simulink library "CRYP_TM_MASTER"  (Simulink 8.6)
settings: Solver=ode45  StartTime=0.0  StopTime=10.0  RelTol=1e-3
libraries: cdsEpicsOut x44, cdsTP x11, cdsFilt x5, cdsFiltCtrl x4, cdsFunctionCall x4, CRYP_TM_MASTER x3, QPD x2, VIS_LIB x1, cdsMuxMatrix x1
(part 1 of 2)
settings Model: Creator=controls  LastModifiedBy=controls

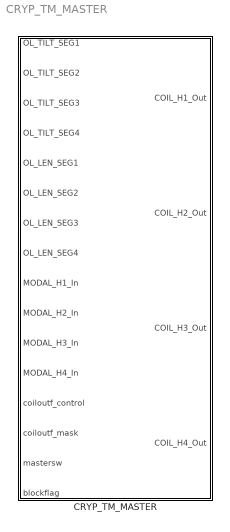
== system CRYP_TM_MASTER ==
  CRYP_TM_MASTER : Subsystem

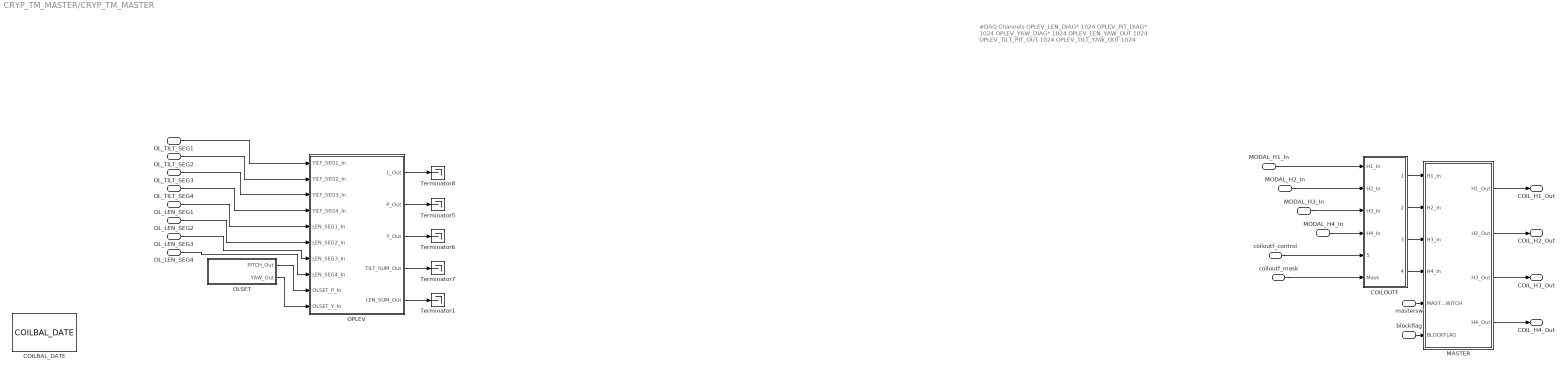
== system CRYP_TM_MASTER/CRYP_TM_MASTER ==
  note: #DAQ Channels
      | OPLEV_LEN_DIAG* 1024
      | OPLEV_PIT_DIAG* 1024
      | OPLEV_YAW_DIAG* 1024
      | OPLEV_LEN_YAW_OUT 1024
      | OPLEV_TILT_PIT_OUT 1024
      | OPLEV_TILT_YAW_OUT 1024
  OL_TILT_SEG1 : Inport
  OL_TILT_SEG2 : Inport  Port=2
  OL_TILT_SEG3 : Inport  Port=3
  OL_TILT_SEG4 : Inport  Port=4
  OL_LEN_SEG1 : Inport  Port=5
  OL_LEN_SEG2 : Inport  Port=6
  OL_LEN_SEG3 : Inport  Port=7
  OL_LEN_SEG4 : Inport  Port=8
  MODAL_H1_In : Inport  Port=9
  MODAL_H2_In : Inport  Port=10
  MODAL_H3_In : Inport  Port=11
  MODAL_H4_In : Inport  Port=12
  coiloutf_control : Inport  Port=13
  coiloutf_mask : Inport  Port=14
  mastersw : Inport  Port=15
  blockflag : Inport  Port=16
  COILBAL_DATE : VIS_LIB/COILBAL_DATE
  COILOUTF : Subsystem
  MASTER : Subsystem
  OLSET : Subsystem
  OPLEV : Subsystem
  Terminator{1,5..8} (5 alike) : Terminator
  COIL_H1_Out : Outport
  COIL_H2_Out : Outport  Port=2
  COIL_H3_Out : Outport  Port=3
  COIL_H4_Out : Outport  Port=4
  wires:
  MODAL_H4_In/1 -> COILOUTF/4(H4_In)
  MODAL_H3_In/1 -> COILOUTF/3(H3_In)
  MODAL_H2_In/1 -> COILOUTF/2(H2_In)
  MODAL_H1_In/1 -> COILOUTF/1(H1_In)
  OL_TILT_SEG3/1 -> OPLEV/3(TILT_SEG3_In)
  OL_LEN_SEG4/1 -> OPLEV/8(LEN_SEG4_In)
  OL_LEN_SEG3/1 -> OPLEV/7(LEN_SEG3_In)
  OL_LEN_SEG2/1 -> OPLEV/6(LEN_SEG2_In)
  OL_LEN_SEG1/1 -> OPLEV/5(LEN_SEG1_In)
  OL_TILT_SEG4/1 -> OPLEV/4(TILT_SEG4_In)
  OL_TILT_SEG2/1 -> OPLEV/2(TILT_SEG2_In)
  OL_TILT_SEG1/1 -> OPLEV/1(TILT_SEG1_In)
  COILOUTF/4(H4_Out) -> MASTER/4(H4_In)
  COILOUTF/3(H3_Out) -> MASTER/3(H3_In)
  COILOUTF/2(H2_Out) -> MASTER/2(H2_In)
  COILOUTF/1(H1_Out) -> MASTER/1(H1_In)
  MASTER/1(H1_Out) -> COIL_H1_Out/1
  MASTER/2(H2_Out) -> COIL_H2_Out/1
  MASTER/3(H3_Out) -> COIL_H3_Out/1
  MASTER/4(H4_Out) -> COIL_H4_Out/1
  OLSET/1(PITCH_Out) -> OPLEV/9(OLSET_P_In)
  OLSET/2(YAW_Out) -> OPLEV/10(OLSET_Y_In)
  coiloutf_control/1 -> COILOUTF/5(Control)
  coiloutf_mask/1 -> COILOUTF/6(Mask)
  mastersw/1 -> MASTER/5(MASTERSWITCH)
  blockflag/1 -> MASTER/6(BLOCKFLAG)
  OPLEV/1(L_Out) -> Terminator8/1
  OPLEV/2(P_Out) -> Terminator5/1
  OPLEV/3(Y_Out) -> Terminator6/1
  OPLEV/4(TILT_SUM_Out) -> Terminator7/1
  OPLEV/5(LEN_SUM_Out) -> Terminator1/1

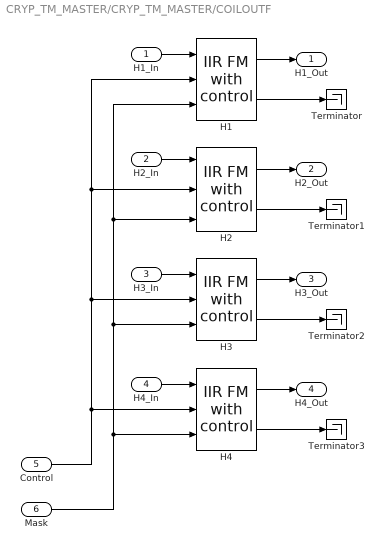
== system CRYP_TM_MASTER/CRYP_TM_MASTER/COILOUTF ==
  H1_In : Inport
  H2_In : Inport  Port=2
  H3_In : Inport  Port=3
  H4_In : Inport  Port=4
  Control : Inport  Port=5
  Mask : Inport  Port=6
  H1 : cdsFiltCtrl/IIR FM with control  Tag=cdsFiltCtrl  Description=|
      | cdsFiltCntrl is the standard IIR filter module (exactly the same as cdsFilt) but with added control data output 'Ctrl'. Filter module digital signal output appears on the first output, which is called 'Val'. 'Ctrl' output has a bit pattern encoding the state of filter's on/off switches (FM1 through FM10). The bit values are:
      |                                                                                                                                                                                                                                                                                                                                       
      | module 	hex	dec                                                                                                                                                                                                                                                                                                                       
      | -----------------------                                                                                                                                                                                                                                                                                                               
      | FM1	0x20                    32                                                                                                                                                                                                                                                                                                        
      | FM2	0x80                     128                                                                                                                                                                                                                                                                                                      
      | FM3	0x200                   512                                                                                                                                                                                                                                                                                                       
      | FM4	0x800                   2048                                                                                                                                                                                                                                                                                                      
      | FM5	0x2000                 8192                                                                                                                                                                                                                                                                                                       
      | FM6	0x8000                 32768                                                                                                                                                                                                                                                                                                      
      | FM7	0x20000                131072                                                                                                                                                                                                                                                                                                     
      | FM8	0x80000                 524288                                                                                                                                                                                                                                                                                                    
      | FM9	0x200000               2097152                                                                                                                                                                                                                                                                                                    
      | FM10	0x800000               8388608                                                                                                                                                                                                                                                                                                   
      |                                                                                                                                                                                                                                                                                                                                       
      | This bit data can be used to drive some other switches or it can be output using a binary I/O module.
      settings: AttributesFormatString=%<Tag>
  H2 : cdsFiltCtrl/IIR FM with control  Tag=cdsFiltCtrl  Description=|
      | cdsFiltCntrl is the standard IIR filter module (exactly the same as cdsFilt) but with added control data output 'Ctrl'. Filter module digital signal output appears on the first output, which is called 'Val'. 'Ctrl' output has a bit pattern encoding the state of filter's on/off switches (FM1 through FM10). The bit values are:
      |                                                                                                                                                                                                                                                                                                                                       
      | module 	hex	dec                                                                                                                                                                                                                                                                                                                       
      | -----------------------                                                                                                                                                                                                                                                                                                               
      | FM1	0x20                    32                                                                                                                                                                                                                                                                                                        
      | FM2	0x80                     128                                                                                                                                                                                                                                                                                                      
      | FM3	0x200                   512                                                                                                                                                                                                                                                                                                       
      | FM4	0x800                   2048                                                                                                                                                                                                                                                                                                      
      | FM5	0x2000                 8192                                                                                                                                                                                                                                                                                                       
      | FM6	0x8000                 32768                                                                                                                                                                                                                                                                                                      
      | FM7	0x20000                131072                                                                                                                                                                                                                                                                                                     
      | FM8	0x80000                 524288                                                                                                                                                                                                                                                                                                    
      | FM9	0x200000               2097152                                                                                                                                                                                                                                                                                                    
      | FM10	0x800000               8388608                                                                                                                                                                                                                                                                                                   
      |                                                                                                                                                                                                                                                                                                                                       
      | This bit data can be used to drive some other switches or it can be output using a binary I/O module.
      settings: AttributesFormatString=%<Tag>
  H3 : cdsFiltCtrl/IIR FM with control  Tag=cdsFiltCtrl  Description=|
      | cdsFiltCntrl is the standard IIR filter module (exactly the same as cdsFilt) but with added control data output 'Ctrl'. Filter module digital signal output appears on the first output, which is called 'Val'. 'Ctrl' output has a bit pattern encoding the state of filter's on/off switches (FM1 through FM10). The bit values are:
      |                                                                                                                                                                                                                                                                                                                                       
      | module 	hex	dec                                                                                                                                                                                                                                                                                                                       
      | -----------------------                                                                                                                                                                                                                                                                                                               
      | FM1	0x20                    32                                                                                                                                                                                                                                                                                                        
      | FM2	0x80                     128                                                                                                                                                                                                                                                                                                      
      | FM3	0x200                   512                                                                                                                                                                                                                                                                                                       
      | FM4	0x800                   2048                                                                                                                                                                                                                                                                                                      
      | FM5	0x2000                 8192                                                                                                                                                                                                                                                                                                       
      | FM6	0x8000                 32768                                                                                                                                                                                                                                                                                                      
      | FM7	0x20000                131072                                                                                                                                                                                                                                                                                                     
      | FM8	0x80000                 524288                                                                                                                                                                                                                                                                                                    
      | FM9	0x200000               2097152                                                                                                                                                                                                                                                                                                    
      | FM10	0x800000               8388608                                                                                                                                                                                                                                                                                                   
      |                                                                                                                                                                                                                                                                                                                                       
      | This bit data can be used to drive some other switches or it can be output using a binary I/O module.
      settings: AttributesFormatString=%<Tag>
  H4 : cdsFiltCtrl/IIR FM with control  Tag=cdsFiltCtrl  Description=|
      | cdsFiltCntrl is the standard IIR filter module (exactly the same as cdsFilt) but with added control data output 'Ctrl'. Filter module digital signal output appears on the first output, which is called 'Val'. 'Ctrl' output has a bit pattern encoding the state of filter's on/off switches (FM1 through FM10). The bit values are:
      |                                                                                                                                                                                                                                                                                                                                       
      | module 	hex	dec                                                                                                                                                                                                                                                                                                                       
      | -----------------------                                                                                                                                                                                                                                                                                                               
      | FM1	0x20                    32                                                                                                                                                                                                                                                                                                        
      | FM2	0x80                     128                                                                                                                                                                                                                                                                                                      
      | FM3	0x200                   512                                                                                                                                                                                                                                                                                                       
      | FM4	0x800                   2048                                                                                                                                                                                                                                                                                                      
      | FM5	0x2000                 8192                                                                                                                                                                                                                                                                                                       
      | FM6	0x8000                 32768                                                                                                                                                                                                                                                                                                      
      | FM7	0x20000                131072                                                                                                                                                                                                                                                                                                     
      | FM8	0x80000                 524288                                                                                                                                                                                                                                                                                                    
      | FM9	0x200000               2097152                                                                                                                                                                                                                                                                                                    
      | FM10	0x800000               8388608                                                                                                                                                                                                                                                                                                   
      |                                                                                                                                                                                                                                                                                                                                       
      | This bit data can be used to drive some other switches or it can be output using a binary I/O module.
      settings: AttributesFormatString=%<Tag>
  Terminator{,1..3} (4 alike) : Terminator
  H1_Out : Outport
  H2_Out : Outport  Port=2
  H3_Out : Outport  Port=3
  H4_Out : Outport  Port=4
  wires:
  H1/1 -> H1_Out/1
  H1_In/1 -> H1/1
  H2_In/1 -> H2/1
  H2/1 -> H2_Out/1
  H3_In/1 -> H3/1
  H3/1 -> H3_Out/1
  H4_In/1 -> H4/1
  H4/1 -> H4_Out/1
  H1/2 -> Terminator/1
  H2/2 -> Terminator1/1
  H4/2 -> Terminator3/1
  H3/2 -> Terminator2/1
  Mask/1 -> H4/3, H3/3, H2/3, H1/3
  Control/1 -> H4/2, H3/2, H2/2, H1/2

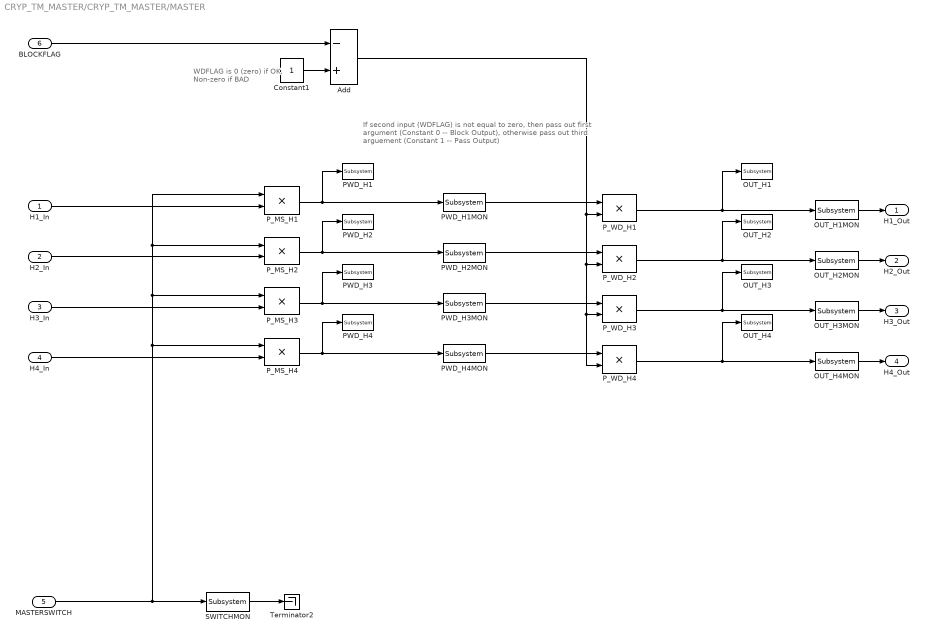
== system CRYP_TM_MASTER/CRYP_TM_MASTER/MASTER ==
  note: WDFLAG is 0 (zero) if OK,
      | Non-zero if BAD
  note: If second input (WDFLAG) is not equal to zero,
      | then pass out first argument (Constant 0 -- Block Output),
      | otherwise pass out third arguement (Constant 1 -- Pass Output)
  H1_In : Inport
  H2_In : Inport  Port=2
  H3_In : Inport  Port=3
  H4_In : Inport  Port=4
  MASTERSWITCH : Inport  Port=5
  BLOCKFLAG : Inport  Port=6
  Add : Sum  Inputs=-+
  Constant1 : Constant
  OUT_H{1..4} (4 alike) : cdsTP/Subsystem  Tag=Test Point
      settings: AttributesFormatString=%<Tag>
  OUT_H1MON : cdsEpicsOut/Subsystem  Tag=cdsEpicsOutput  Description=|
      | Purpose:                                          
      | Output a FE signal to an EPICS channel.           
      |                                                   
      | Operation:                                        
      | Takes input value and passes it to EPICS record.  
      |                                                   
      | Usage:                                            
      | Name the part with the desired EPICS rrecord name.
      settings: AttributesFormatString=%<Tag>
  OUT_H2MON : cdsEpicsOut/Subsystem  Tag=cdsEpicsOutput  Description=|
      | Purpose:                                          
      | Output a FE signal to an EPICS channel.           
      |                                                   
      | Operation:                                        
      | Takes input value and passes it to EPICS record.  
      |                                                   
      | Usage:                                            
      | Name the part with the desired EPICS rrecord name.
      settings: AttributesFormatString=%<Tag>
  OUT_H3MON : cdsEpicsOut/Subsystem  Tag=cdsEpicsOutput  Description=|
      | Purpose:                                          
      | Output a FE signal to an EPICS channel.           
      |                                                   
      | Operation:                                        
      | Takes input value and passes it to EPICS record.  
      |                                                   
      | Usage:                                            
      | Name the part with the desired EPICS rrecord name.
      settings: AttributesFormatString=%<Tag>
  OUT_H4MON : cdsEpicsOut/Subsystem  Tag=cdsEpicsOutput  Description=|
      | Purpose:                                          
      | Output a FE signal to an EPICS channel.           
      |                                                   
      | Operation:                                        
      | Takes input value and passes it to EPICS record.  
      |                                                   
      | Usage:                                            
      | Name the part with the desired EPICS rrecord name.
      settings: AttributesFormatString=%<Tag>
  PWD_H{1..4} (4 alike) : cdsTP/Subsystem  Tag=Test Point
      settings: AttributesFormatString=%<Tag>
  PWD_H1MON : cdsEpicsOut/Subsystem  Tag=cdsEpicsOutput  Description=|
      | Purpose:                                          
      | Output a FE signal to an EPICS channel.           
      |                                                   
      | Operation:                                        
      | Takes input value and passes it to EPICS record.  
      |                                                   
      | Usage:                                            
      | Name the part with the desired EPICS rrecord name.
      settings: AttributesFormatString=%<Tag>
  PWD_H2MON : cdsEpicsOut/Subsystem  Tag=cdsEpicsOutput  Description=|
      | Purpose:                                          
      | Output a FE signal to an EPICS channel.           
      |                                                   
      | Operation:                                        
      | Takes input value and passes it to EPICS record.  
      |                                                   
      | Usage:                                            
      | Name the part with the desired EPICS rrecord name.
      settings: AttributesFormatString=%<Tag>
  PWD_H3MON : cdsEpicsOut/Subsystem  Tag=cdsEpicsOutput  Description=|
      | Purpose:                                          
      | Output a FE signal to an EPICS channel.           
      |                                                   
      | Operation:                                        
      | Takes input value and passes it to EPICS record.  
      |                                                   
      | Usage:                                            
      | Name the part with the desired EPICS rrecord name.
      settings: AttributesFormatString=%<Tag>
  PWD_H4MON : cdsEpicsOut/Subsystem  Tag=cdsEpicsOutput  Description=|
      | Purpose:                                          
      | Output a FE signal to an EPICS channel.           
      |                                                   
      | Operation:                                        
      | Takes input value and passes it to EPICS record.  
      |                                                   
      | Usage:                                            
      | Name the part with the desired EPICS rrecord name.
      settings: AttributesFormatString=%<Tag>
  P_MS_H{1..4} (4 alike) : Product  RndMeth=Zero
  P_WD_H{1..4} (4 alike) : Product  RndMeth=Zero
  SWITCHMON : cdsEpicsOut/Subsystem  Tag=cdsEpicsOutput  Description=|
      | Purpose:                                          
      | Output a FE signal to an EPICS channel.           
      |                                                   
      | Operation:                                        
      | Takes input value and passes it to EPICS record.  
      |                                                   
      | Usage:                                            
      | Name the part with the desired EPICS rrecord name.
      settings: AttributesFormatString=%<Tag>
  Terminator2 : Terminator
  H1_Out : Outport
  H2_Out : Outport  Port=2
  H3_Out : Outport  Port=3
  H4_Out : Outport  Port=4
  wires:
  SWITCHMON/1 -> Terminator2/1
  BLOCKFLAG/1 -> Add/1
  Constant1/1 -> Add/2
  P_WD_H4/1 -> OUT_H4/1, OUT_H4MON/1
  P_WD_H3/1 -> OUT_H3/1, OUT_H3MON/1
  P_WD_H2/1 -> OUT_H2/1, OUT_H2MON/1
  P_WD_H1/1 -> OUT_H1/1, OUT_H1MON/1
  P_MS_H4/1 -> PWD_H4/1, PWD_H4MON/1
  P_MS_H3/1 -> PWD_H3/1, PWD_H3MON/1
  P_MS_H2/1 -> PWD_H2/1, PWD_H2MON/1
  P_MS_H1/1 -> PWD_H1/1, PWD_H1MON/1
  OUT_H4MON/1 -> H4_Out/1
  OUT_H3MON/1 -> H3_Out/1
  OUT_H1MON/1 -> H1_Out/1
  OUT_H2MON/1 -> H2_Out/1
  MASTERSWITCH/1 -> SWITCHMON/1, P_MS_H1/1, P_MS_H2/1, P_MS_H3/1, P_MS_H4/1
  H4_In/1 -> P_MS_H4/2
  H3_In/1 -> P_MS_H3/2
  H2_In/1 -> P_MS_H2/2
  H1_In/1 -> P_MS_H1/2
  PWD_H1MON/1 -> P_WD_H1/1
  PWD_H2MON/1 -> P_WD_H2/1
  PWD_H3MON/1 -> P_WD_H3/1
  PWD_H4MON/1 -> P_WD_H4/1
  Add/1 -> P_WD_H4/2, P_WD_H3/2, P_WD_H2/2, P_WD_H1/2

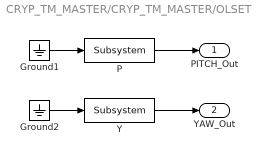
== system CRYP_TM_MASTER/CRYP_TM_MASTER/OLSET ==
  Ground1 : Ground
  Ground2 : Ground
  P : cdsFilt/Subsystem  Tag=cdsFilt  Description=|
      | Purpose:                                                                                                                                                                                                                                  
      | Standard CDS IIR filter module.                                                                                                                                                                                                           
      |                                                                                                                                                                                                                                           
      | Operation:                                                                                                                                                                                                                                
      | Consists of 10 second order section IIR filters, plus a ramped gain stage. In FE code, also provides pre-defined test points and excitation channel inputs. The filter coefficients are defined in the LIGO system using the 'foton' tool.
      |                                                                                                                                                                                                                                           
      | Usage:                                                                                                                                                                                                                                    
      | Name the part with the desired filter module name.
      settings: AttributesFormatString=%<Tag>
  Y : cdsFilt/Subsystem  Tag=cdsFilt  Description=|
      | Purpose:                                                                                                                                                                                                                                  
      | Standard CDS IIR filter module.                                                                                                                                                                                                           
      |                                                                                                                                                                                                                                           
      | Operation:                                                                                                                                                                                                                                
      | Consists of 10 second order section IIR filters, plus a ramped gain stage. In FE code, also provides pre-defined test points and excitation channel inputs. The filter coefficients are defined in the LIGO system using the 'foton' tool.
      |                                                                                                                                                                                                                                           
      | Usage:                                                                                                                                                                                                                                    
      | Name the part with the desired filter module name.
      settings: AttributesFormatString=%<Tag>
  PITCH_Out : Outport
  YAW_Out : Outport  Port=2
  wires:
  P/1 -> PITCH_Out/1
  Y/1 -> YAW_Out/1
  Ground1/1 -> P/1
  Ground2/1 -> Y/1

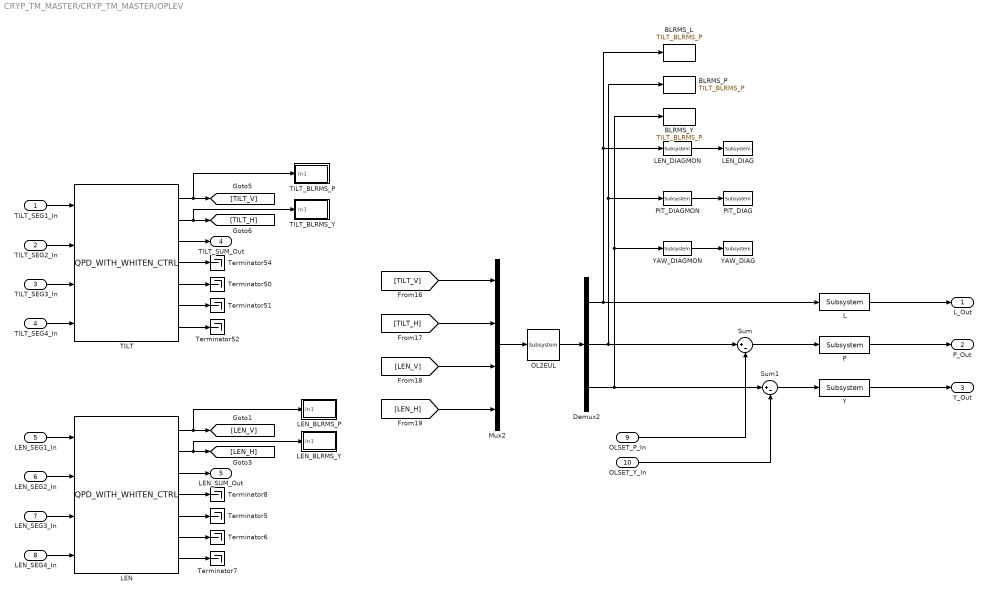
== system CRYP_TM_MASTER/CRYP_TM_MASTER/OPLEV ==
  TILT_SEG1_In : Inport
  TILT_SEG2_In : Inport  Port=2
  TILT_SEG3_In : Inport  Port=3
  TILT_SEG4_In : Inport  Port=4
  LEN_SEG1_In : Inport  Port=5
  LEN_SEG2_In : Inport  Port=6
  LEN_SEG3_In : Inport  Port=7
  LEN_SEG4_In : Inport  Port=8
  OLSET_P_In : Inport  Port=9
  OLSET_Y_In : Inport  Port=10
  BLRMS_L : CRYP_TM_MASTER/CRYP_TM_MASTER/OPLEV/TILT_BLRMS_P
  BLRMS_P : CRYP_TM_MASTER/CRYP_TM_MASTER/OPLEV/TILT_BLRMS_P
  BLRMS_Y : CRYP_TM_MASTER/CRYP_TM_MASTER/OPLEV/TILT_BLRMS_P
  Demux2 : Demux  Outputs=3
  L : cdsFilt/Subsystem  Tag=cdsFilt  Description=|
      | Purpose:                                                                                                                                                                                                                                  
      | Standard CDS IIR filter module.                                                                                                                                                                                                           
      |                                                                                                                                                                                                                                           
      | Operation:                                                                                                                                                                                                                                
      | Consists of 10 second order section IIR filters, plus a ramped gain stage. In FE code, also provides pre-defined test points and excitation channel inputs. The filter coefficients are defined in the LIGO system using the 'foton' tool.
      |                                                                                                                                                                                                                                           
      | Usage:                                                                                                                                                                                                                                    
      | Name the part with the desired filter module name.
      settings: AttributesFormatString=%<Tag>
  LEN : QPD/QPD_WITH_WHITEN_CTRL
  LEN_BLRMS_P : Subsystem
  LEN_BLRMS_Y : Subsystem
  LEN_DIAG : cdsTP/Subsystem  Tag=Test Point
      settings: AttributesFormatString=%<Tag>
  LEN_DIAGMON : cdsEpicsOut/Subsystem  Tag=cdsEpicsOutput  Description=|
      | Purpose:                                          
      | Output a FE signal to an EPICS channel.           
      |                                                   
      | Operation:                                        
      | Takes input value and passes it to EPICS record.  
      |                                                   
      | Usage:                                            
      | Name the part with the desired EPICS rrecord name.
      settings: AttributesFormatString=%<Tag>
  Mux2 : Mux
  OL2EUL : cdsMuxMatrix/Subsystem  Tag=cdsMuxMatrix  Description=Any size matrix. Inputs and outputs must be connected using Mux and Demux parts.
      settings: AttributesFormatString=%<Tag>
  P : cdsFilt/Subsystem  Tag=cdsFilt  Description=|
      | Purpose:                                                                                                                                                                                                                                  
      | Standard CDS IIR filter module.                                                                                                                                                                                                           
      |                                                                                                                                                                                                                                           
      | Operation:                                                                                                                                                                                                                                
      | Consists of 10 second order section IIR filters, plus a ramped gain stage. In FE code, also provides pre-defined test points and excitation channel inputs. The filter coefficients are defined in the LIGO system using the 'foton' tool.
      |                                                                                                                                                                                                                                           
      | Usage:                                                                                                                                                                                                                                    
      | Name the part with the desired filter module name.
      settings: AttributesFormatString=%<Tag>
  PIT_DIAG : cdsTP/Subsystem  Tag=Test Point
      settings: AttributesFormatString=%<Tag>
  PIT_DIAGMON : cdsEpicsOut/Subsystem  Tag=cdsEpicsOutput  Description=|
      | Purpose:                                          
      | Output a FE signal to an EPICS channel.           
      |                                                   
      | Operation:                                        
      | Takes input value and passes it to EPICS record.  
      |                                                   
      | Usage:                                            
      | Name the part with the desired EPICS rrecord name.
      settings: AttributesFormatString=%<Tag>
  Sum : Sum  Inputs=|+-
  Sum1 : Sum  Inputs=|+-
  TILT : QPD/QPD_WITH_WHITEN_CTRL
  TILT_BLRMS_P : Subsystem
  TILT_BLRMS_Y : Subsystem
  Terminator{5..8,50..52,54} (8 alike) : Terminator
  Y : cdsFilt/Subsystem  Tag=cdsFilt  Description=|
      | Purpose:                                                                                                                                                                                                                                  
      | Standard CDS IIR filter module.                                                                                                                                                                                                           
      |                                                                                                                                                                                                                                           
      | Operation:                                                                                                                                                                                                                                
      | Consists of 10 second order section IIR filters, plus a ramped gain stage. In FE code, also provides pre-defined test points and excitation channel inputs. The filter coefficients are defined in the LIGO system using the 'foton' tool.
      |                                                                                                                                                                                                                                           
      | Usage:                                                                                                                                                                                                                                    
      | Name the part with the desired filter module name.
      settings: AttributesFormatString=%<Tag>
  YAW_DIAG : cdsTP/Subsystem  Tag=Test Point
      settings: AttributesFormatString=%<Tag>
  YAW_DIAGMON : cdsEpicsOut/Subsystem  Tag=cdsEpicsOutput  Description=|
      | Purpose:                                          
      | Output a FE signal to an EPICS channel.           
      |                                                   
      | Operation:                                        
      | Takes input value and passes it to EPICS record.  
      |                                                   
      | Usage:                                            
      | Name the part with the desired EPICS rrecord name.
      settings: AttributesFormatString=%<Tag>
  L_Out : Outport
  P_Out : Outport  Port=2
  Y_Out : Outport  Port=3
  TILT_SUM_Out : Outport  Port=4
  LEN_SUM_Out : Outport  Port=5
  wires:
  [TILT_H] -> Mux2/2
  Demux2/3 -> Sum1/1, BLRMS_Y/1, YAW_DIAGMON/1
  LEN/4 -> Terminator8/1
  LEN/5 -> Terminator5/1
  LEN/6 -> Terminator6/1
  LEN/7 -> Terminator7/1
  [TILT_V] -> Mux2/1
  LEN_SEG4_In/1 -> LEN/4
  LEN/2 -> [LEN_H], LEN_BLRMS_Y/1(In1)
  LEN/1 -> [LEN_V], LEN_BLRMS_P/1(In1)
  LEN/3 -> LEN_SUM_Out/1
  [LEN_V] -> Mux2/3
  LEN_SEG1_In/1 -> LEN/1
  LEN_SEG2_In/1 -> LEN/2
  LEN_SEG3_In/1 -> LEN/3
  OL2EUL/1 -> Demux2/1
  TILT_SEG1_In/1 -> TILT/1
  TILT_SEG2_In/1 -> TILT/2
  TILT_SEG3_In/1 -> TILT/3
  TILT_SEG4_In/1 -> TILT/4
  TILT/2 -> TILT_BLRMS_Y/1(In1), [TILT_H]
  TILT/1 -> TILT_BLRMS_P/1(In1), [TILT_V]
  TILT/3 -> TILT_SUM_Out/1
  TILT/4 -> Terminator54/1
  TILT/6 -> Terminator51/1
  TILT/7 -> Terminator52/1
  TILT/5 -> Terminator50/1
  Demux2/2 -> Sum/1, BLRMS_P/1, PIT_DIAGMON/1
  Mux2/1 -> OL2EUL/1
  [LEN_H] -> Mux2/4
  P/1 -> P_Out/1
  Y/1 -> Y_Out/1
  Demux2/1 -> L/1, BLRMS_L/1, LEN_DIAGMON/1
  YAW_DIAGMON/1 -> YAW_DIAG/1
  PIT_DIAGMON/1 -> PIT_DIAG/1
  LEN_DIAGMON/1 -> LEN_DIAG/1
  L/1 -> L_Out/1
  Sum/1 -> P/1
  Sum1/1 -> Y/1
  OLSET_P_In/1 -> Sum/2
  OLSET_Y_In/1 -> Sum1/2
